simulink model "WTG"  (R2021a)
settings: Solver=VariableStepAuto  StartTime=0.0  StopTime=10.0  RelTol=1e-3
values from neighbouring files (symbols this model uses):
  cCpTabCpDataV126 = [0.003 0.0041 0.0052 0.0062 0.0072 0.0082 0.0092 0.0101 0.0111 0.012 0.013 0.014 ... (910 elements, 26x35)]    [cptabcpdataV126.mat]
  cCpTabLambdaBinsV126 = [1 1.5 2 2.5 3 3.5 4 4.5 5 5.5 6 6.5 ... (35 elements, 1x35)]    [cptablambdaV126.mat]
  cCpTabPitchPosBinsV126 = [-4 -2 0 2 4 6 8 10 12 14 16 18 ... (26 elements, 1x26)]    [cptabpitchposV126.mat]
  cCtTabCpDataV126 = [0.0546 0.0541 0.0535 0.0528 0.0521 0.0513 0.0505 0.0497 0.0488 0.0479 0.047 0.0461 ... (910 elements, 26x35)]    [cttabcpdataV126.mat]
  cCtTabLambdaBinsV126 = [1 1.5 2 2.5 3 3.5 4 4.5 5 5.5 6 6.5 ... (35 elements, 1x35)]    [cttablambdaV126.mat]
  cCtTabPitchPosBinsV126 = [-4 -2 0 2 4 6 8 10 12 14 16 18 ... (26 elements, 1x26)]    [cttabpitchposV126.mat]
undefined symbols (not defined in the file or in its folder): rad, s
libraries: aerolibconvert2 x1
settings Model: Creator=Chitra Manis Raja  LastModifiedBy=Chitra Manis Raja

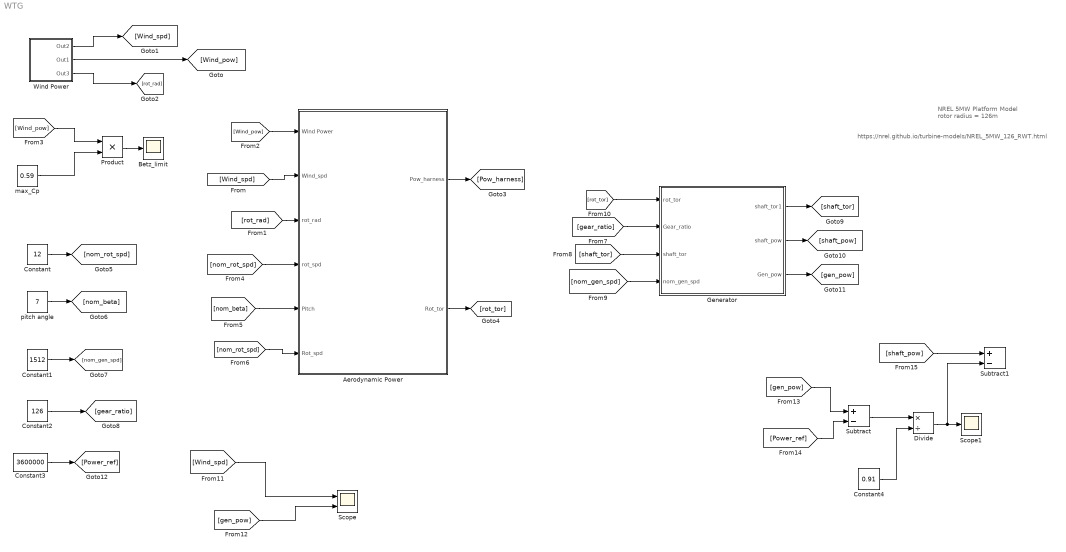
== system WTG ==
  note: https://nrel.github.io/turbine-models/NREL_5MW_126_RWT.html
  note: NREL 5MW Platform Model
      | rotor radius = 126m
  Aerodynamic Power : Subsystem
  Betz_limit : Scope
  Constant : Constant  Value=12
  Constant1 : Constant  Value=1512
  Constant2 : Constant  Value=126
  Constant3 : Constant  Value=3600000
  Constant4 : Constant  Value=0.91
  Divide : Product  Inputs=*/
  Generator : Subsystem
  Product : Product
  Scope : Scope  NumInputPorts=2
  Scope1 : Scope
  Subtract : Sum  Inputs=+-
  Subtract1 : Sum  Inputs=+-
  Wind Power : Subsystem
  max_Cp : Constant  Value=0.59
  pitch angle : Constant  Value=7
  wires:
  Wind Power/2(Out1) -> [Wind_pow]
  max_Cp/1 -> Product/2
  Product/1 -> Betz_limit/1
  Wind Power/3(Out3) -> [rot_rad]
  Wind Power/1(Out2) -> [Wind_spd]
  [Wind_pow] -> Product/1
  Constant/1 -> [nom_rot_spd]
  pitch angle/1 -> [nom_beta]
  Constant1/1 -> [nom_gen_spd]
  Constant2/1 -> [gear_ratio]
  Aerodynamic Power/2(Rot_tor) -> [rot_tor]
  [Wind_pow] -> Aerodynamic Power/1(Wind Power)
  [Wind_spd] -> Aerodynamic Power/2(Wind_spd)
  [rot_rad] -> Aerodynamic Power/3(rot_rad)
  [nom_rot_spd] -> Aerodynamic Power/4(rot_spd)
  [nom_beta] -> Aerodynamic Power/5(Pitch)
  [nom_rot_spd] -> Aerodynamic Power/6(Rot_spd)
  Aerodynamic Power/1(Pow_harness) -> [Pow_harness]
  [rot_tor] -> Generator/1(rot_tor)
  [gear_ratio] -> Generator/2(Gear_ratio)
  [shaft_tor] -> Generator/3(shaft_tor)
  [nom_gen_spd] -> Generator/4(nom_gen_spd)
  Generator/1(shaft_tor1) -> [shaft_tor]
  Generator/2(shaft_pow) -> [shaft_pow]
  Generator/3(Gen_pow) -> [gen_pow]
  [Wind_spd] -> Scope/1
  [gen_pow] -> Scope/2
  Constant3/1 -> [Power_ref]
  [gen_pow] -> Subtract/1
  [Power_ref] -> Subtract/2
  Subtract/1 -> Divide/1
  Constant4/1 -> Divide/2
  Divide/1 -> Subtract1/2, Scope1/1
  [shaft_pow] -> Subtract1/1

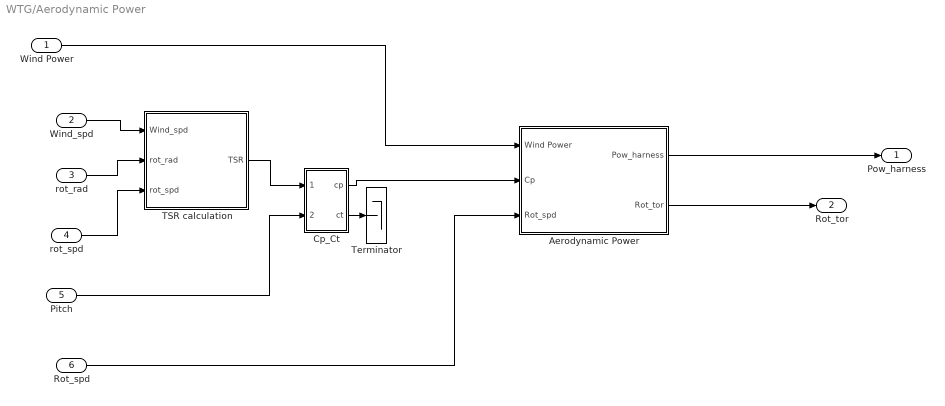
== system WTG/Aerodynamic Power ==
  Wind Power : Inport
  Wind_spd : Inport  Port=2
  rot_rad : Inport  Port=3
  rot_spd : Inport  Port=4
  Pitch : Inport  Port=5
  Rot_spd : Inport  Port=6
  Aerodynamic Power : Subsystem
  Cp_Ct : Subsystem
  TSR calculation : Subsystem
  Terminator : Terminator
  Pow_harness : Outport
  Rot_tor : Outport  Port=2
  wires:
  rot_rad/1 -> TSR calculation/2(rot_rad)
  rot_spd/1 -> TSR calculation/3(rot_spd)
  Wind Power/1 -> Aerodynamic Power/1(Wind Power)
  TSR calculation/1(TSR) -> Cp_Ct/1(TSR)
  Cp_Ct/1(cp) -> Aerodynamic Power/2(Cp)
  Cp_Ct/2(ct) -> Terminator/1
  Pitch/1 -> Cp_Ct/2(Pitch)
  Wind_spd/1 -> TSR calculation/1(Wind_spd)
  Aerodynamic Power/1(Pow_harness) -> Pow_harness/1
  Aerodynamic Power/2(Rot_tor) -> Rot_tor/1
  Rot_spd/1 -> Aerodynamic Power/3(Rot_spd)

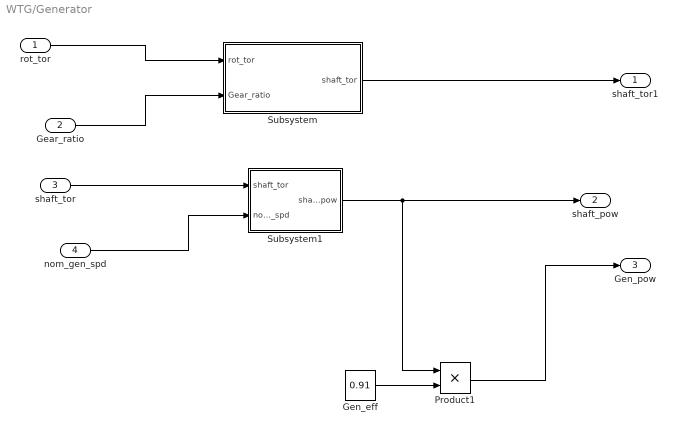
== system WTG/Generator ==
  rot_tor : Inport
  Gear_ratio : Inport  Port=2
  shaft_tor : Inport  Port=3
  nom_gen_spd : Inport  Port=4
  Gen_eff : Constant  Value=0.91
  Product1 : Product
  Subsystem : Subsystem
  Subsystem1 : Subsystem
  shaft_tor1 : Outport
  shaft_pow : Outport  Port=2
  Gen_pow : Outport  Port=3
  wires:
  shaft_tor/1 -> Subsystem1/1(shaft_tor)
  Gen_eff/1 -> Product1/2
  nom_gen_spd/1 -> Subsystem1/2(nom_gen_spd)
  Subsystem1/1(shaft_pow) -> shaft_pow/1, Product1/1
  Gear_ratio/1 -> Subsystem/2(Gear_ratio)
  Subsystem/1(shaft_tor) -> shaft_tor1/1
  rot_tor/1 -> Subsystem/1(rot_tor)
  Product1/1 -> Gen_pow/1

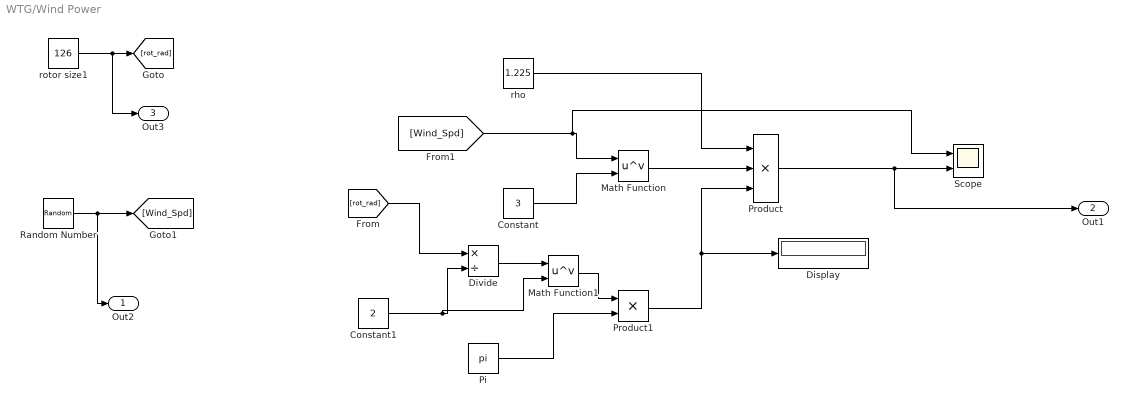
== system WTG/Wind Power ==
  Constant : Constant  Value=3
  Constant1 : Constant  Value=2
  Display : Display
  Divide : Product  Inputs=*/
  Math Function : Math  Operator=pow  SaturateOnIntegerOverflow=on
  Math Function1 : Math  Operator=pow  SaturateOnIntegerOverflow=on
  Pi : Constant  Value=pi  OutDataTypeStr=Inherit: Inherit via back propagation
  Product : Product  Inputs=3
  Product1 : Product
  Random Number : RandomNumber  Mean=10  SampleTime=0.1
  Scope : Scope  NumInputPorts=2
  rho : Constant  Value=1.225
  rotor size1 : Constant  Value=126
  Out2 : Outport
  Out1 : Outport  Port=2
  Out3 : Outport  Port=3
  wires:
  Constant/1 -> Math Function/2
  Divide/1 -> Math Function1/1
  [rot_rad] -> Divide/1
  [Wind_Spd] -> Scope/1, Math Function/1
  Product/1 -> Out1/1, Scope/2
  Product1/1 -> Product/3, Display/1
  rho/1 -> Product/1
  Constant1/1 -> Math Function1/2, Divide/2
  Math Function/1 -> Product/2
  Pi/1 -> Product1/2
  Math Function1/1 -> Product1/1
  rotor size1/1 -> Out3/1, [rot_rad]
  Random Number/1 -> Out2/1, [Wind_Spd]

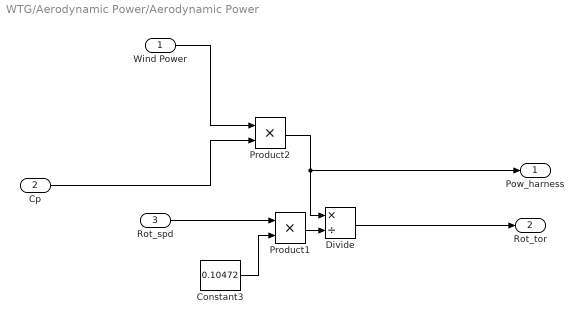
== system WTG/Aerodynamic Power/Aerodynamic Power ==
  Wind Power : Inport
  Cp : Inport  Port=2
  Rot_spd : Inport  Port=3
  Constant3 : Constant  Value=0.10472
  Divide : Product  Inputs=*/
  Product1 : Product
  Product2 : Product
  Pow_harness : Outport
  Rot_tor : Outport  Port=2
  wires:
  Constant3/1 -> Product1/2
  Product1/1 -> Divide/2
  Product2/1 -> Pow_harness/1, Divide/1
  Cp/1 -> Product2/2
  Wind Power/1 -> Product2/1
  Rot_spd/1 -> Product1/1
  Divide/1 -> Rot_tor/1

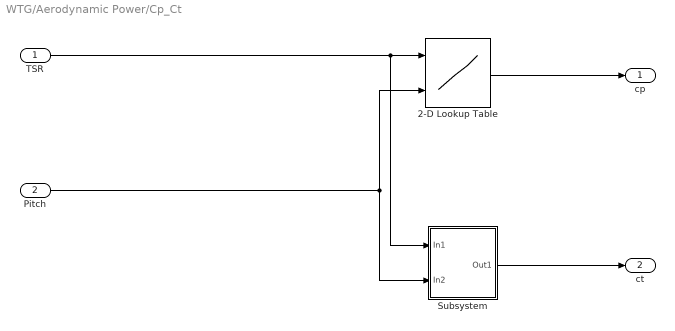
== system WTG/Aerodynamic Power/Cp_Ct ==
  TSR : Inport
  Pitch : Inport  Port=2
  2-D Lookup Table : Lookup_n-D  BreakpointsForDimension1=cCpTabPitchPosBinsV126  BreakpointsForDimension2=cCpTabLambdaBinsV126  Table=cCpTabCpDataV126  RndMeth=Simplest  InputSameDT=on
      settings: InputPortMap=u0,u1
  Subsystem : Subsystem
  cp : Outport
  ct : Outport  Port=2
  wires:
  Pitch/1 -> 2-D Lookup Table/2, Subsystem/2(In2)
  Subsystem/1(Out1) -> ct/1
  TSR/1 -> Subsystem/1(In1), 2-D Lookup Table/1
  2-D Lookup Table/1 -> cp/1

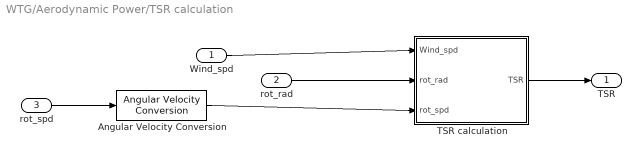
== system WTG/Aerodynamic Power/TSR calculation ==
  Wind_spd : Inport
  rot_rad : Inport  Port=2
  rot_spd : Inport  Port=3
  Angular Velocity Conversion : aerolibconvert2/Angular Velocity Conversion  IU=rpm  OU=rad/s
  TSR calculation : MATLAB Function  TreatAsAtomicUnit=on
  TSR : Outport
  wires:
  TSR calculation/1(TSR) -> TSR/1
  Angular Velocity Conversion/1 -> TSR calculation/3(rot_spd)
  rot_rad/1 -> TSR calculation/2(rot_rad)
  rot_spd/1 -> Angular Velocity Conversion/1
  Wind_spd/1 -> TSR calculation/1(Wind_spd)

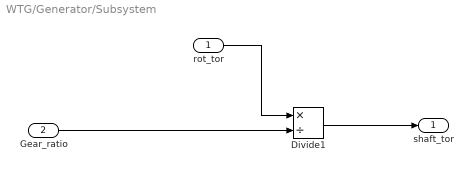
== system WTG/Generator/Subsystem ==
  rot_tor : Inport
  Gear_ratio : Inport  Port=2
  Divide1 : Product  Inputs=*/
  shaft_tor : Outport
  wires:
  rot_tor/1 -> Divide1/1
  Divide1/1 -> shaft_tor/1
  Gear_ratio/1 -> Divide1/2

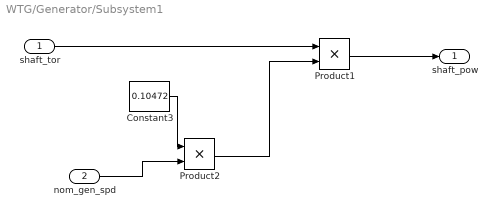
== system WTG/Generator/Subsystem1 ==
  shaft_tor : Inport
  nom_gen_spd : Inport  Port=2
  Constant3 : Constant  Value=0.10472
  Product1 : Product
  Product2 : Product
  shaft_pow : Outport
  wires:
  Product2/1 -> Product1/2
  shaft_tor/1 -> Product1/1
  Constant3/1 -> Product2/1
  nom_gen_spd/1 -> Product2/2
  Product1/1 -> shaft_pow/1

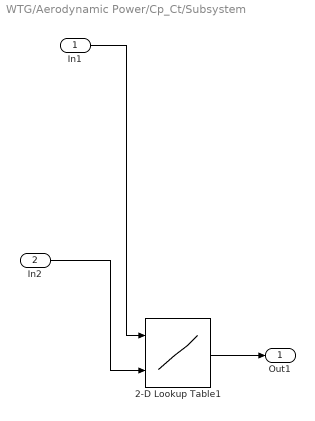
== system WTG/Aerodynamic Power/Cp_Ct/Subsystem ==
  In1 : Inport
  In2 : Inport  Port=2
  2-D Lookup Table1 : Lookup_n-D  BreakpointsForDimension1=cCtTabPitchPosBinsV126  BreakpointsForDimension2=cCtTabLambdaBinsV126  Table=cCtTabCpDataV126  RndMeth=Simplest  InputSameDT=on
      settings: InputPortMap=u0,u1
  Out1 : Outport
  wires:
  In2/1 -> 2-D Lookup Table1/2
  2-D Lookup Table1/1 -> Out1/1
  In1/1 -> 2-D Lookup Table1/1

== matlab function WTG/Aerodynamic Power/TSR calculation/TSR calculation ==
  data: Wind_spd input; TSR output; rot_rad input; rot_spd input
function TSR = fcn(Wind_spd,rot_rad,rot_spd)
omega=rot_spd*0.5 %omega => angular velocity
TSR = omega*rot_rad/Wind_spd; %omega*rot_rad = speed of rotor tip
